simulink model "example1"  (R2024b)
settings: Solver=FixedStepAuto  StartTime=0.0  StopTime=20  FixedStep=0.001  RelTol=1e-3
(part 1 of 3)
settings Model: Creator=aqx  LastModifiedBy=aqx
settings ModelReferenceCC: EnableRefExpFcnMdlSchedulingChecks=on
settings RTWCC: GPUComputeCapability=3.5

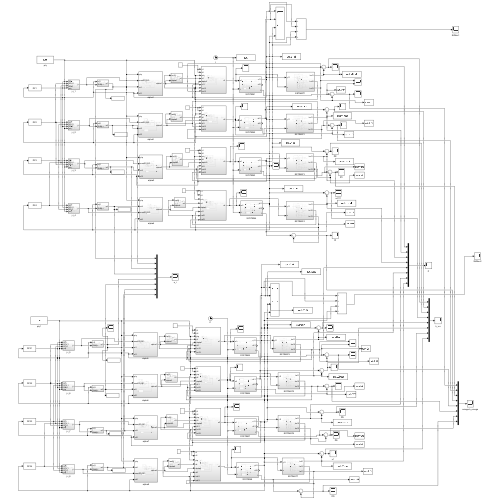
[thumbnail: Simulink's stored preview of the top-level diagram]
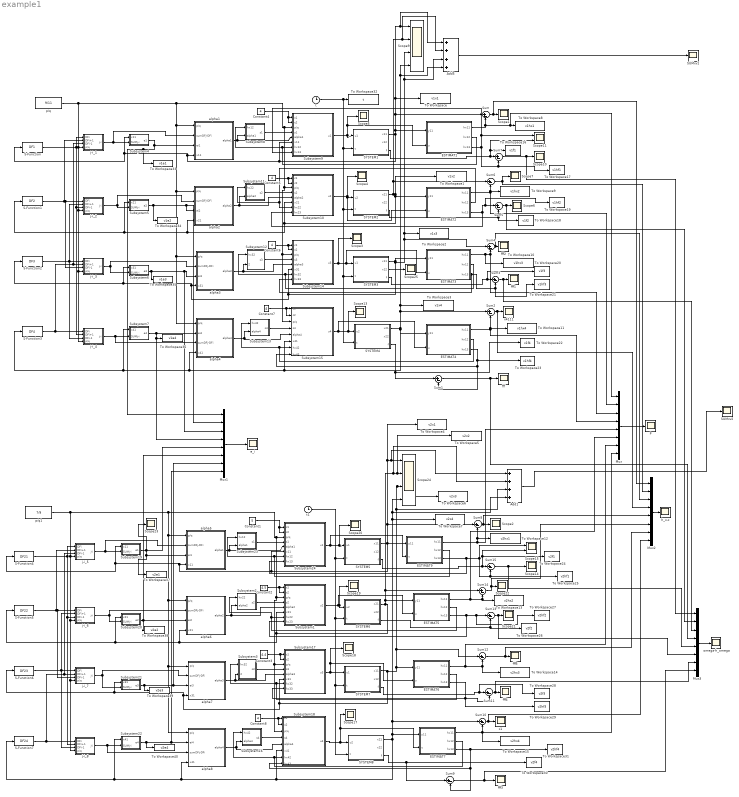
== system example1 ==
  Add1 : Sum  Inputs=4
  Add5 : Sum  Inputs=4
  Constant1 : Constant  Value=5
  Constant2 : Constant  Value=4.5
  Constant3 : Constant  Value=4.4
  Constant{4..8} (5 alike) : Constant  Value=4
  ESTIMAT1 : Subsystem
  ESTIMAT2 : Subsystem
  ESTIMAT3 : Subsystem
  ESTIMAT4 : Subsystem
  ESTIMAT5 : Subsystem
  ESTIMAT6 : Subsystem
  ESTIMAT7 : Subsystem
  ESTIMAT9 : Subsystem
  Mux{,1..3} (4 alike) : Mux  Inputs=8
  P : Scope
  S-Function : S-Function  FunctionName=DF1  SFunctionDeploymentMode=off  EnableBusSupport=off
  S-Function1 : S-Function  FunctionName=DF2  SFunctionDeploymentMode=off  EnableBusSupport=off
  S-Function2 : S-Function  FunctionName=DF3  SFunctionDeploymentMode=off  EnableBusSupport=off
  S-Function3 : S-Function  FunctionName=DF4  SFunctionDeploymentMode=off  EnableBusSupport=off
  S-Function4 : S-Function  FunctionName=DF21  SFunctionDeploymentMode=off  EnableBusSupport=off
  S-Function5 : S-Function  FunctionName=DF22  SFunctionDeploymentMode=off  EnableBusSupport=off
  S-Function6 : S-Function  FunctionName=DF23  SFunctionDeploymentMode=off  EnableBusSupport=off
  S-Function7 : S-Function  FunctionName=DF24  SFunctionDeploymentMode=off  EnableBusSupport=off
  SUMxv1 : Scope
  SUMxv2 : Scope
  SYSTEM1 : Subsystem
  SYSTEM2 : Subsystem
  SYSTEM3 : Subsystem
  SYSTEM4 : Subsystem
  SYSTEM5 : Subsystem
  SYSTEM6 : Subsystem
  SYSTEM7 : Subsystem
  SYSTEM8 : Subsystem
  Scope{1..7,10,13..14,17..23,25} (18 alike) : Scope
  Scope11 : Scope  NumInputPorts=2
  Scope15 : Scope  NumInputPorts=2
  Scope24 : Scope  NumInputPorts=4
  Scope9 : Scope  NumInputPorts=4
  Subsystem1 : Subsystem
  Subsystem10 : Subsystem
  Subsystem11 : Subsystem
  Subsystem12 : Subsystem
  Subsystem13 : Subsystem
  Subsystem14 : Subsystem
  Subsystem15 : Subsystem
  Subsystem16 : Subsystem
  Subsystem17 : Subsystem
  Subsystem18 : Subsystem
  Subsystem19 : Subsystem
  Subsystem2 : Subsystem
  Subsystem20 : Subsystem
  Subsystem21 : Subsystem
  Subsystem22 : Subsystem
  Subsystem23 : Subsystem
  Subsystem24 : Subsystem
  Subsystem3 : Subsystem
  Subsystem4 : Subsystem
  Subsystem5 : Subsystem
  Subsystem6 : Subsystem
  Subsystem7 : Subsystem
  Subsystem8 : Subsystem
  Subsystem9 : Subsystem
  Sum{,1..15} (16 alike) : Sum  Inputs=|+-
  To Workspace : ToWorkspace  VariableName=v1x1  SampleTime=-1
  To Workspace1 : ToWorkspace  VariableName=v1x2  SampleTime=-1
  To Workspace10 : ToWorkspace  VariableName=v1hx3  SampleTime=-1
  To Workspace11 : ToWorkspace  VariableName=v1hx4  SampleTime=-1
  To Workspace12 : ToWorkspace  VariableName=v2hx1  SampleTime=-1
  To Workspace13 : ToWorkspace  VariableName=v2hx2  SampleTime=-1
  To Workspace14 : ToWorkspace  VariableName=v2hx3  SampleTime=-1
  To Workspace15 : ToWorkspace  VariableName=v2hx4  SampleTime=-1
  To Workspace16 : ToWorkspace  VariableName=v1f1  SampleTime=-1
  To Workspace17 : ToWorkspace  VariableName=v1hf1  SampleTime=-1
  To Workspace18 : ToWorkspace  VariableName=v1f2  SampleTime=-1
  To Workspace19 : ToWorkspace  VariableName=v1hf2  SampleTime=-1
  To Workspace2 : ToWorkspace  VariableName=v1x3  SampleTime=-1
  To Workspace20 : ToWorkspace  VariableName=v1f3  SampleTime=-1
  To Workspace21 : ToWorkspace  VariableName=v1hf3  SampleTime=-1
  To Workspace22 : ToWorkspace  VariableName=v1f4  SampleTime=-1
  To Workspace23 : ToWorkspace  VariableName=v1hf4  SampleTime=-1
  To Workspace24 : ToWorkspace  VariableName=v2f1  SampleTime=-1
  To Workspace25 : ToWorkspace  VariableName=v2hf1  SampleTime=-1
  To Workspace26 : ToWorkspace  VariableName=v2f2  SampleTime=-1
  To Workspace27 : ToWorkspace  VariableName=v2hf2  SampleTime=-1
  To Workspace28 : ToWorkspace  VariableName=v2f3  SampleTime=-1
  To Workspace29 : ToWorkspace  VariableName=v2hf3  SampleTime=-1
  To Workspace3 : ToWorkspace  VariableName=v1x4  SampleTime=-1
  To Workspace30 : ToWorkspace  VariableName=v2f4  SampleTime=-1
  To Workspace31 : ToWorkspace  VariableName=v2hf4  SampleTime=-1
  To Workspace32 : ToWorkspace  VariableName=t  SampleTime=-1
  To Workspace33 : ToWorkspace  VariableName=v1e1  SampleTime=-1
  To Workspace34 : ToWorkspace  VariableName=v1e2  SampleTime=-1
  To Workspace35 : ToWorkspace  VariableName=v1e3  SampleTime=-1
  To Workspace36 : ToWorkspace  VariableName=v1e4  SampleTime=-1
  To Workspace37 : ToWorkspace  VariableName=v2e1  SampleTime=-1
  To Workspace38 : ToWorkspace  VariableName=v2e2  SampleTime=-1
  To Workspace39 : ToWorkspace  VariableName=v2e3  SampleTime=-1
  To Workspace4 : ToWorkspace  VariableName=v2x1  SampleTime=-1
  To Workspace40 : ToWorkspace  VariableName=v2e4  SampleTime=-1
  To Workspace5 : ToWorkspace  VariableName=v2x2  SampleTime=-1
  To Workspace6 : ToWorkspace  VariableName=v2x3  SampleTime=-1
  To Workspace7 : ToWorkspace  VariableName=v2x4  SampleTime=-1
  To Workspace8 : ToWorkspace  VariableName=v1hx1  SampleTime=-1
  To Workspace9 : ToWorkspace  VariableName=v1hx2  SampleTime=-1
  alpha1 : Subsystem
  alpha2 : Subsystem
  alpha3 : Subsystem
  alpha4 : Subsystem
  alpha5 : Subsystem
  alpha6 : Subsystem
  alpha7 : Subsystem
  alpha8 : Subsystem
  e_i : Scope
  fff{,1..5} (6 alike) : Scope
  h_x-x : Scope
  j-i_1 : Subsystem
  j-i_2 : Subsystem
  j-i_3 : Subsystem
  j-i_4 : Subsystem
  j-i_5 : Subsystem
  j-i_6 : Subsystem
  j-i_7 : Subsystem
  j-i_8 : Subsystem
  omega-h_omega : Scope
  p/q : Constant  Value=9/11
  p/q1 : Constant  Value=7/9
  t : Clock
  t1 : Clock
  x1 : Scope
  x4111 : Scope
  wires:
  S-Function/1 -> j-i_4/2(DFi+1), j-i_2/3(DFi-1), j-i_1/1(DFi)
  S-Function1/1 -> j-i_3/3(DFi-1), j-i_2/1(DFi), j-i_1/2(DFi+1)
  S-Function3/1 -> j-i_3/2(DFi+1), j-i_1/3(DFi-1), j-i_4/1(DFi)
  S-Function2/1 -> j-i_2/2(DFi+1), j-i_4/3(DFi-1), j-i_3/1(DFi)
  j-i_1/1(j-i) -> Subsystem4/2(SUMj-i), alpha1/2(sumDFj-DFi)
  j-i_2/1(j-i) -> alpha2/2(sumDFj-DFi), Subsystem5/2(SUMj-i)
  j-i_3/1(j-i) -> Subsystem6/2(SUMj-i), alpha3/2(sumDFj-DFi)
  j-i_4/1(j-i) -> alpha4/3(sumDFj-DFi), Subsystem7/2(SUMj-i)
  Subsystem4/1(e1) -> Mux1/1, To Workspace33/1, alpha1/3(ei1)
  Subsystem5/1(e2) -> To Workspace34/1, Mux1/2, alpha2/3(ei2)
  Subsystem6/1(e3) -> To Workspace35/1, Mux1/3, alpha3/3(ei3)
  Subsystem7/1(e4) -> Mux1/4, To Workspace36/1, alpha4/2(ei4)
  p/q/1 -> j-i_4/4(p/q), j-i_3/4(p/q), j-i_2/4(p/q), j-i_1/4(p/q), alpha4/1(p/q), alpha3/1(p/q), alpha2/1(p/q), alpha1/1(p/q), Subsystem15/3(p/q), Subsystem14/3(p/q), Subsystem10/3(p/q), Subsystem9/3(p/q)
  alpha1/1(alpha1) -> Subsystem8/2(alpha1), Subsystem9/5(alpha1)
  Subsystem8/1(s1) -> Subsystem9/4(s1)
  alpha2/1(alpha2) -> Subsystem10/5(alpha2), Subsystem11/2(alpha2)
  Subsystem11/1(s2) -> Subsystem10/4(s2)
  alpha3/1(alpha3) -> Subsystem12/2(alpha3), Subsystem14/5(alpha3)
  alpha4/1(alpha4) -> Subsystem15/5(alpha4), Subsystem13/2(alpha4)
  Subsystem12/1(s3) -> Subsystem14/4(s3)
  Subsystem13/1(s4) -> Subsystem15/4(s4)
  Subsystem14/1(u3) -> ESTIMAT3/2(u), SYSTEM3/1(u1), Scope3/1
  Subsystem15/1(u4) -> ESTIMAT4/2(u), Scope13/1, SYSTEM4/1(u2)
  Constant4/1 -> Subsystem9/2(c2), Subsystem9/1(c1)
  Subsystem9/1(u1) -> ESTIMAT1/2(u), Scope5/1, SYSTEM1/1(u1)
  Subsystem10/1(u2) -> ESTIMAT2/2(u), SYSTEM2/1(u2), Scope4/1
  Constant5/1 -> Subsystem10/2(c2), Subsystem10/1(c1)
  Constant6/1 -> Subsystem14/2(c2), Subsystem14/1(c1)
  Constant7/1 -> Subsystem15/2(c2), Subsystem15/1(c1)
  SYSTEM1/1(x11) -> To Workspace/1, Add5/1, Scope9/1, Sum/1, ESTIMAT1/1(y11), S-Function/1, Subsystem4/1(x11), alpha1/4(x11), Subsystem9/6(x11)
  SYSTEM2/1(x21) -> Add5/2, Scope9/2, Sum6/1, ESTIMAT2/1(y11), S-Function1/1, Subsystem5/1(x21), alpha2/4(x21), Subsystem10/6(x21), To Workspace1/1
  SYSTEM3/1(x11) -> Subsystem14/6(x31), S-Function2/1, Subsystem6/1(x31), alpha3/4(x31), To Workspace2/1, Scope9/3, Add5/3, Sum4/1, ESTIMAT3/1(y11)
  SYSTEM4/1(x21) -> ESTIMAT4/1(y11), Subsystem15/6(x41), S-Function3/1, Subsystem7/1(x41), alpha4/4(x41), Scope9/4, Add5/4, To Workspace3/1, Sum2/1
  Sum/1 -> Mux2/1, Scope1/1
  SYSTEM4/3(f) -> Sum1/1, To Workspace22/1
  Sum1/1 -> Mux3/4, fff/1
  Sum2/1 -> Mux2/4, x4111/1
  SYSTEM3/3(f) -> To Workspace20/1, Sum3/1
  Sum3/1 -> Mux3/3, fff1/1
  Sum4/1 -> Mux2/3, fff2/1
  SYSTEM2/3(f) -> To Workspace18/1, Sum5/2
  Sum5/1 -> Mux3/2, Scope6/1
  Sum6/1 -> Mux2/2, Scope7/1
  SYSTEM1/3(f) -> Scope11/2, To Workspace16/1, Sum7/1
  Sum7/1 -> Mux3/1, Scope10/1
  Add5/1 -> SUMxv1/1
  Subsystem20/1(e2) -> To Workspace38/1, Mux1/6, alpha6/3(ei2)
  Subsystem19/1(e1) -> Mux1/5, To Workspace37/1, alpha5/3(ei1), Scope23/1
  Subsystem22/1(e4) -> Mux1/8, alpha8/2(ei4), To Workspace40/1
  S-Function4/1 -> j-i_8/2(DFi+1), j-i_6/3(DFi-1), j-i_5/1(DFi)
  S-Function5/1 -> j-i_7/3(DFi-1), j-i_6/1(DFi), j-i_5/2(DFi+1)
  Sum11/1 -> Mux3/7, fff4/1
  SYSTEM7/3(f) -> To Workspace28/1, Sum11/1
  Subsystem16/1(s4) -> Subsystem18/4(s4)
  ESTIMAT7/2(hx12) -> Subsystem16/1(hx42), Subsystem18/7(hx42)
  ESTIMAT7/1(hx11) -> Mux/8, To Workspace15/1, Sum10/2
  S-Function7/1 -> j-i_7/2(DFi+1), j-i_5/3(DFi-1), j-i_8/1(DFi)
  SYSTEM8/3(f) -> To Workspace30/1, Sum9/1
  j-i_6/1(j-i) -> alpha6/2(sumDFj-DFi), Subsystem20/2(SUMj-i)
  ESTIMAT9/1(hx11) -> Mux/5, Sum8/2, To Workspace12/1
  alpha5/1(alpha1) -> Subsystem23/2(alpha1), Subsystem24/5(alpha1)
  Sum8/1 -> Mux2/5, Scope2/1
  ESTIMAT7/3(hx13) -> Sum9/2, Subsystem18/8(hx43), To Workspace31/1
  Constant1/1 -> Subsystem24/2(c2), Subsystem24/1(c1)
  ESTIMAT6/3(hx13) -> Sum11/2, Subsystem17/8(hx33), To Workspace29/1
  SYSTEM7/1(x11) -> ESTIMAT6/1(y11), To Workspace6/1, Scope24/3, Add1/3, Sum12/1, Subsystem17/6(x31), S-Function6/1, Subsystem21/1(x31), alpha7/4(x31)
  ESTIMAT6/2(hx12) -> Subsystem3/1(hx32), Subsystem17/7(hx32)
  ESTIMAT5/2(hx12) -> Subsystem2/1(hx22), Subsystem1/7(hx22)
  Subsystem21/1(e3) -> Mux1/7, alpha7/3(ei3), To Workspace39/1
  Constant3/1 -> Subsystem17/2(c2), Subsystem17/1(c1)
  SYSTEM5/1(x11) -> ESTIMAT9/1(y11), To Workspace4/1, Add1/1, Scope24/1, Sum8/1, S-Function4/1, Subsystem19/1(x11), alpha5/4(x11), Subsystem24/6(x11)
  t1/1 -> SYSTEM8/2(t), SYSTEM7/2(t), SYSTEM6/2(t), SYSTEM5/2(t)
  SYSTEM6/1(x21) -> ESTIMAT5/1(y11), Add1/2, To Workspace5/1, Scope24/2, Sum14/1, S-Function5/1, Subsystem20/1(x21), alpha6/4(x21), Subsystem1/6(x21)
  Constant8/1 -> Subsystem18/2(c2), Subsystem18/1(c1)
  Constant2/1 -> Subsystem1/2(c2), Subsystem1/1(c1)
  Subsystem18/1(u4) -> ESTIMAT7/2(u), Scope17/1, SYSTEM8/1(u2)
  j-i_8/1(j-i) -> alpha8/3(sumDFj-DFi), Subsystem22/2(SUMj-i)
  j-i_5/1(j-i) -> Subsystem19/2(SUMj-i), alpha5/2(sumDFj-DFi)
  Subsystem17/1(u3) -> SYSTEM7/1(u1), ESTIMAT6/2(u), Scope18/1
  Subsystem3/1(s3) -> Subsystem17/4(s3)
  alpha8/1(alpha4) -> Subsystem18/5(alpha4), Subsystem16/2(alpha4)
  alpha7/1(alpha3) -> Subsystem3/2(alpha3), Subsystem17/5(alpha3)
  alpha6/1(alpha2) -> Subsystem1/5(alpha2), Subsystem2/2(alpha2)
  p/q1/1 -> j-i_8/4(p/q), j-i_7/4(p/q), j-i_6/4(p/q), j-i_5/4(p/q), alpha8/1(p/q), alpha7/1(p/q), alpha6/1(p/q), alpha5/1(p/q), Subsystem18/3(p/q), Subsystem17/3(p/q), Subsystem1/3(p/q), Subsystem24/3(p/q)
  ESTIMAT6/1(hx11) -> Mux/7, To Workspace14/1, Sum12/2
  Subsystem2/1(s2) -> Subsystem1/4(s2)
  Sum9/1 -> Mux3/8, fff3/1
  SYSTEM5/3(f) -> Scope15/2, To Workspace24/1, Sum15/1
  j-i_7/1(j-i) -> Subsystem21/2(SUMj-i), alpha7/2(sumDFj-DFi)
  Sum10/1 -> Mux2/8, x1/1
  Sum15/1 -> Mux3/5, Scope14/1
  SYSTEM8/1(x21) -> ESTIMAT7/1(y11), Scope24/4, Add1/4, To Workspace7/1, Sum10/1, Subsystem18/6(x41), S-Function7/1, Subsystem22/1(x41), alpha8/4(x41)
  Add1/1 -> SUMxv2/1
  Sum12/1 -> Mux2/7, fff5/1
  ESTIMAT9/3(hx13) -> Subsystem24/8(hx13), To Workspace25/1, Sum15/2, Scope15/1
  S-Function6/1 -> j-i_6/2(DFi+1), j-i_8/3(DFi-1), j-i_7/1(DFi)
  Sum13/1 -> Mux3/6, Scope21/1
  Subsystem1/1(u2) -> ESTIMAT5/2(u), Scope19/1, SYSTEM6/1(u2)
  Subsystem24/1(u1) -> ESTIMAT9/2(u), SYSTEM5/1(u1), Scope20/1
  Sum14/1 -> Mux2/6, Scope22/1
  Subsystem23/1(s1) -> Subsystem24/4(s1)
  ESTIMAT5/1(hx11) -> Mux/6, To Workspace13/1, Sum14/2
  ESTIMAT5/3(hx13) -> To Workspace27/1, Sum13/1, Subsystem1/8(hx23)
  SYSTEM6/3(f) -> Sum13/2, To Workspace26/1
  ESTIMAT9/2(hx12) -> Subsystem23/1(hx12), Subsystem24/7(hx12)
  t/1 -> To Workspace32/1, SYSTEM4/2(t), SYSTEM3/2(t), SYSTEM2/2(t), SYSTEM1/2(t)
  ESTIMAT1/1(hx11) -> Sum/2, Mux/1, To Workspace8/1
  ESTIMAT1/3(hx13) -> Subsystem9/8(hx13), Scope11/1, To Workspace17/1, Sum7/2
  ESTIMAT1/2(hx12) -> Subsystem8/1(hx12), Subsystem9/7(hx12)
  ESTIMAT2/1(hx11) -> Mux/2, To Workspace9/1, Sum6/2
  ESTIMAT2/3(hx13) -> Subsystem10/8(hx23), To Workspace19/1, Sum5/1
  ESTIMAT2/2(hx12) -> Subsystem10/7(hx22), Subsystem11/1(hx22)
  ESTIMAT3/1(hx11) -> To Workspace10/1, Mux/3, Sum4/2
  ESTIMAT3/3(hx13) -> Subsystem14/8(hx33), To Workspace21/1, Sum3/2
  ESTIMAT3/2(hx12) -> Subsystem12/1(hx32), Subsystem14/7(hx32)
  ESTIMAT4/1(hx11) -> Sum2/2, To Workspace11/1, Mux/4
  ESTIMAT4/3(hx13) -> To Workspace23/1, Subsystem15/8(hx43), Sum1/2
  ESTIMAT4/2(hx12) -> Subsystem13/1(hx42), Subsystem15/7(hx42)
  SYSTEM3/2(x12) -> Scope25/1
  Mux/1 -> P/1
  Mux1/1 -> e_i/1
  Mux2/1 -> h_x-x/1
  Mux3/1 -> omega-h_omega/1

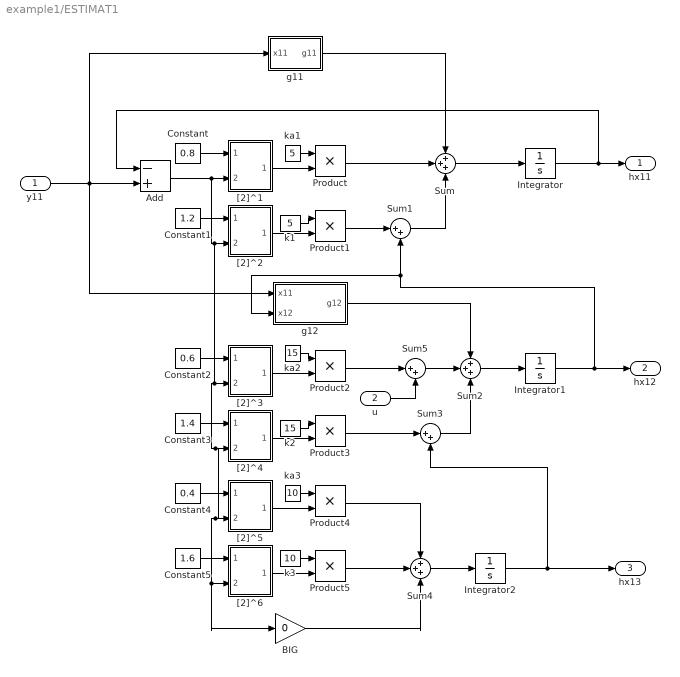
== system example1/ESTIMAT1 ==
  y11 : Inport
  u : Inport  Port=2
  Add : Sum  Inputs=-+
  BIG : Gain  Gain=0
  Constant : Constant  Value=0.8
  Constant1 : Constant  Value=1.2
  Constant2 : Constant  Value=0.6
  Constant3 : Constant  Value=1.4
  Constant4 : Constant  Value=0.4
  Constant5 : Constant  Value=1.6
  Integrator : Integrator  InitialCondition=1
  Integrator1 : Integrator  InitialCondition=1
  Integrator2 : Integrator  InitialCondition=1
  Product{,1..5} (6 alike) : Product
  Sum : Sum  Inputs=3
  Sum1 : Sum  Inputs=|++
  Sum2 : Sum  Inputs=3
  Sum3 : Sum  Inputs=|++
  Sum4 : Sum  Inputs=3
  Sum5 : Sum  Inputs=|++
  "[2]^1" : Subsystem
  "[2]^2" : Subsystem
  "[2]^3" : Subsystem
  "[2]^4" : Subsystem
  "[2]^5" : Subsystem
  "[2]^6" : Subsystem
  g11 : Subsystem
  g12 : Subsystem
  k1 : Constant  Value=5
  k2 : Constant  Value=15
  k3 : Constant  Value=10
  ka1 : Constant  Value=5
  ka2 : Constant  Value=15
  ka3 : Constant  Value=10
  hx11 : Outport
  hx12 : Outport  Port=2
  hx13 : Outport  Port=3
  wires:
  Integrator/1 -> Add/1, hx11/1
  Sum1/1 -> Sum/3
  Sum/1 -> Integrator/1
  Integrator1/1 -> g12/2(x12), Sum1/2, hx12/1
  y11/1 -> g12/1(x11), g11/1(x11), Add/2
  "[2]^1"/1(Out1) -> Product/2
  "[2]^2"/1(Out1) -> Product1/2
  ka1/1 -> Product/1
  k1/1 -> Product1/1
  g11/1(g11) -> Sum/1
  Product/1 -> Sum/2
  Product1/1 -> Sum1/1
  Sum2/1 -> Integrator1/1
  Sum3/1 -> Sum2/3
  Integrator2/1 -> hx13/1, Sum3/2
  g12/1(g12) -> Sum2/1
  ka2/1 -> Product2/1
  k2/1 -> Product3/1
  "[2]^4"/1(Out1) -> Product3/2
  "[2]^3"/1(Out1) -> Product2/2
  Product3/1 -> Sum3/1
  Sum4/1 -> Integrator2/1
  k3/1 -> Product5/1
  "[2]^6"/1(Out1) -> Product5/2
  ka3/1 -> Product4/1
  Add/1 -> BIG/1, "[2]^6"/2(In2), "[2]^5"/2(In2), "[2]^4"/2(In2), "[2]^3"/2(In2), "[2]^2"/2(In2), "[2]^1"/2(In2)
  "[2]^5"/1(Out1) -> Product4/2
  Product5/1 -> Sum4/2
  Product4/1 -> Sum4/1
  BIG/1 -> Sum4/3
  Product2/1 -> Sum5/1
  Sum5/1 -> Sum2/2
  u/1 -> Sum5/2
  Constant/1 -> "[2]^1"/1(In1)
  Constant1/1 -> "[2]^2"/1(beta1)
  Constant2/1 -> "[2]^3"/1(In1)
  Constant3/1 -> "[2]^4"/1(beta1)
  Constant4/1 -> "[2]^5"/1(In1)
  Constant5/1 -> "[2]^6"/1(beta1)

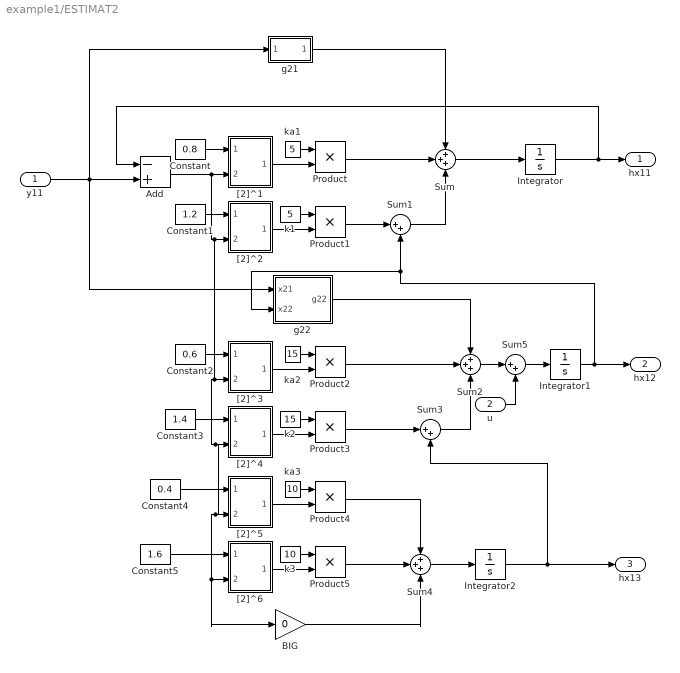
== system example1/ESTIMAT2 ==
  y11 : Inport
  u : Inport  Port=2
  Add : Sum  Inputs=-+
  BIG : Gain  Gain=0
  Constant : Constant  Value=0.8
  Constant1 : Constant  Value=1.2
  Constant2 : Constant  Value=0.6
  Constant3 : Constant  Value=1.4
  Constant4 : Constant  Value=0.4
  Constant5 : Constant  Value=1.6
  Integrator : Integrator  InitialCondition=3
  Integrator1 : Integrator  InitialCondition=1
  Integrator2 : Integrator  InitialCondition=1
  Product{,1..5} (6 alike) : Product
  Sum : Sum  Inputs=3
  Sum1 : Sum  Inputs=|++
  Sum2 : Sum  Inputs=3
  Sum3 : Sum  Inputs=|++
  Sum4 : Sum  Inputs=3
  Sum5 : Sum  Inputs=|++
  "[2]^1" : Subsystem
  "[2]^2" : Subsystem
  "[2]^3" : Subsystem
  "[2]^4" : Subsystem
  "[2]^5" : Subsystem
  "[2]^6" : Subsystem
  g21 : Subsystem
  g22 : Subsystem
  k1 : Constant  Value=5
  k2 : Constant  Value=15
  k3 : Constant  Value=10
  ka1 : Constant  Value=5
  ka2 : Constant  Value=15
  ka3 : Constant  Value=10
  hx11 : Outport
  hx12 : Outport  Port=2
  hx13 : Outport  Port=3
  wires:
  Integrator/1 -> Add/1, hx11/1
  Sum1/1 -> Sum/3
  Sum/1 -> Integrator/1
  Integrator1/1 -> g22/2(x22), Sum1/2, hx12/1
  y11/1 -> g22/1(x21), g21/1(x21), Add/2
  "[2]^1"/1(Out1) -> Product/2
  "[2]^2"/1(Out1) -> Product1/2
  ka1/1 -> Product/1
  k1/1 -> Product1/1
  g21/1(g21) -> Sum/1
  Product/1 -> Sum/2
  Product1/1 -> Sum1/1
  Sum3/1 -> Sum2/3
  Integrator2/1 -> hx13/1, Sum3/2
  g22/1(g22) -> Sum2/1
  ka2/1 -> Product2/1
  k2/1 -> Product3/1
  "[2]^4"/1(Out1) -> Product3/2
  "[2]^3"/1(Out1) -> Product2/2
  Product2/1 -> Sum2/2
  Product3/1 -> Sum3/1
  Sum4/1 -> Integrator2/1
  k3/1 -> Product5/1
  "[2]^6"/1(Out1) -> Product5/2
  ka3/1 -> Product4/1
  Add/1 -> BIG/1, "[2]^6"/2(In2), "[2]^5"/2(In2), "[2]^4"/2(In2), "[2]^3"/2(In2), "[2]^2"/2(In2), "[2]^1"/2(In2)
  "[2]^5"/1(Out1) -> Product4/2
  Product5/1 -> Sum4/2
  Product4/1 -> Sum4/1
  BIG/1 -> Sum4/3
  Sum2/1 -> Sum5/1
  Sum5/1 -> Integrator1/1
  u/1 -> Sum5/2
  Constant/1 -> "[2]^1"/1(In1)
  Constant1/1 -> "[2]^2"/1(beta1)
  Constant2/1 -> "[2]^3"/1(In1)
  Constant3/1 -> "[2]^4"/1(beta1)
  Constant4/1 -> "[2]^5"/1(In1)
  Constant5/1 -> "[2]^6"/1(beta1)

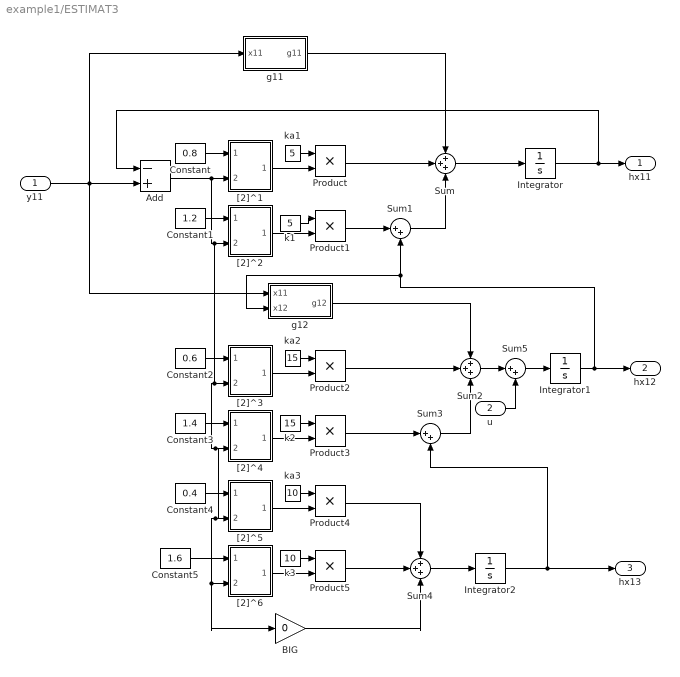
== system example1/ESTIMAT3 ==
  y11 : Inport
  u : Inport  Port=2
  Add : Sum  Inputs=-+
  BIG : Gain  Gain=0
  Constant : Constant  Value=0.8
  Constant1 : Constant  Value=1.2
  Constant2 : Constant  Value=0.6
  Constant3 : Constant  Value=1.4
  Constant4 : Constant  Value=0.4
  Constant5 : Constant  Value=1.6
  Integrator : Integrator  InitialCondition=1
  Integrator1 : Integrator  InitialCondition=1
  Integrator2 : Integrator  InitialCondition=1
  Product{,1..5} (6 alike) : Product
  Sum : Sum  Inputs=3
  Sum1 : Sum  Inputs=|++
  Sum2 : Sum  Inputs=3
  Sum3 : Sum  Inputs=|++
  Sum4 : Sum  Inputs=3
  Sum5 : Sum  Inputs=|++
  "[2]^1" : Subsystem
  "[2]^2" : Subsystem
  "[2]^3" : Subsystem
  "[2]^4" : Subsystem
  "[2]^5" : Subsystem
  "[2]^6" : Subsystem
  g11 : Subsystem
  g12 : Subsystem
  k1 : Constant  Value=5
  k2 : Constant  Value=15
  k3 : Constant  Value=10
  ka1 : Constant  Value=5
  ka2 : Constant  Value=15
  ka3 : Constant  Value=10
  hx11 : Outport
  hx12 : Outport  Port=2
  hx13 : Outport  Port=3
  wires:
  Integrator/1 -> Add/1, hx11/1
  Sum1/1 -> Sum/3
  Sum/1 -> Integrator/1
  Integrator1/1 -> g12/2(x12), Sum1/2, hx12/1
  y11/1 -> g12/1(x11), g11/1(x11), Add/2
  "[2]^1"/1(Out1) -> Product/2
  "[2]^2"/1(Out1) -> Product1/2
  ka1/1 -> Product/1
  k1/1 -> Product1/1
  g11/1(g11) -> Sum/1
  Product/1 -> Sum/2
  Product1/1 -> Sum1/1
  Sum3/1 -> Sum2/3
  Integrator2/1 -> hx13/1, Sum3/2
  g12/1(g12) -> Sum2/1
  ka2/1 -> Product2/1
  k2/1 -> Product3/1
  "[2]^4"/1(Out1) -> Product3/2
  "[2]^3"/1(Out1) -> Product2/2
  Product2/1 -> Sum2/2
  Product3/1 -> Sum3/1
  Sum4/1 -> Integrator2/1
  k3/1 -> Product5/1
  "[2]^6"/1(Out1) -> Product5/2
  ka3/1 -> Product4/1
  Add/1 -> BIG/1, "[2]^6"/2(In2), "[2]^5"/2(In2), "[2]^4"/2(In2), "[2]^3"/2(In2), "[2]^2"/2(In2), "[2]^1"/2(In2)
  "[2]^5"/1(Out1) -> Product4/2
  Product5/1 -> Sum4/2
  Product4/1 -> Sum4/1
  BIG/1 -> Sum4/3
  Sum2/1 -> Sum5/1
  Sum5/1 -> Integrator1/1
  u/1 -> Sum5/2
  Constant/1 -> "[2]^1"/1(In1)
  Constant1/1 -> "[2]^2"/1(beta1)
  Constant2/1 -> "[2]^3"/1(In1)
  Constant3/1 -> "[2]^4"/1(beta1)
  Constant4/1 -> "[2]^5"/1(In1)
  Constant5/1 -> "[2]^6"/1(beta1)

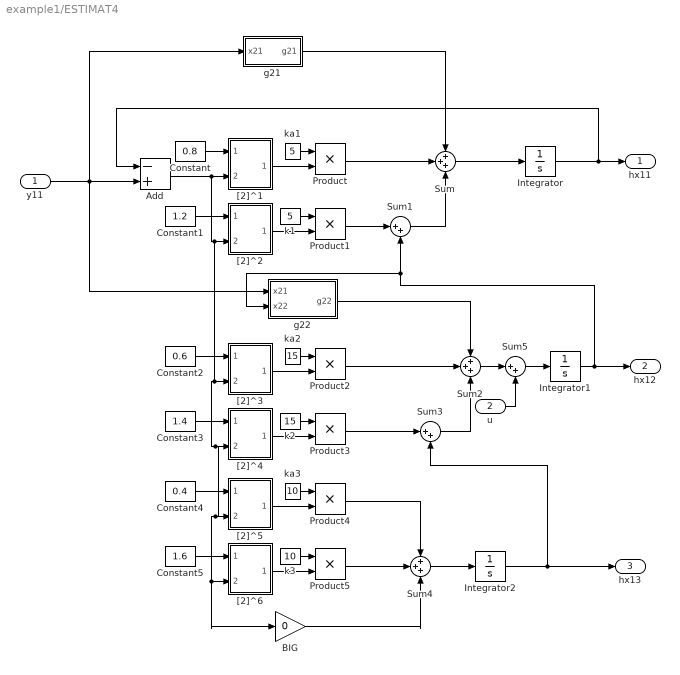
== system example1/ESTIMAT4 ==
  y11 : Inport
  u : Inport  Port=2
  Add : Sum  Inputs=-+
  BIG : Gain  Gain=0
  Constant : Constant  Value=0.8
  Constant1 : Constant  Value=1.2
  Constant2 : Constant  Value=0.6
  Constant3 : Constant  Value=1.4
  Constant4 : Constant  Value=0.4
  Constant5 : Constant  Value=1.6
  Integrator : Integrator  InitialCondition=5
  Integrator1 : Integrator  InitialCondition=1
  Integrator2 : Integrator  InitialCondition=1
  Product{,1..5} (6 alike) : Product
  Sum : Sum  Inputs=3
  Sum1 : Sum  Inputs=|++
  Sum2 : Sum  Inputs=3
  Sum3 : Sum  Inputs=|++
  Sum4 : Sum  Inputs=3
  Sum5 : Sum  Inputs=|++
  "[2]^1" : Subsystem
  "[2]^2" : Subsystem
  "[2]^3" : Subsystem
  "[2]^4" : Subsystem
  "[2]^5" : Subsystem
  "[2]^6" : Subsystem
  g21 : Subsystem
  g22 : Subsystem
  k1 : Constant  Value=5
  k2 : Constant  Value=15
  k3 : Constant  Value=10
  ka1 : Constant  Value=5
  ka2 : Constant  Value=15
  ka3 : Constant  Value=10
  hx11 : Outport
  hx12 : Outport  Port=2
  hx13 : Outport  Port=3
  wires:
  Integrator/1 -> Add/1, hx11/1
  Sum1/1 -> Sum/3
  Sum/1 -> Integrator/1
  Integrator1/1 -> g22/2(x22), Sum1/2, hx12/1
  y11/1 -> g22/1(x21), g21/1(x21), Add/2
  "[2]^1"/1(Out1) -> Product/2
  "[2]^2"/1(Out1) -> Product1/2
  ka1/1 -> Product/1
  k1/1 -> Product1/1
  g21/1(g21) -> Sum/1
  Product/1 -> Sum/2
  Product1/1 -> Sum1/1
  Sum3/1 -> Sum2/3
  Integrator2/1 -> hx13/1, Sum3/2
  g22/1(g22) -> Sum2/1
  ka2/1 -> Product2/1
  k2/1 -> Product3/1
  "[2]^4"/1(Out1) -> Product3/2
  "[2]^3"/1(Out1) -> Product2/2
  Product2/1 -> Sum2/2
  Product3/1 -> Sum3/1
  Sum4/1 -> Integrator2/1
  k3/1 -> Product5/1
  "[2]^6"/1(Out1) -> Product5/2
  ka3/1 -> Product4/1
  Add/1 -> BIG/1, "[2]^6"/2(In2), "[2]^5"/2(In2), "[2]^4"/2(In2), "[2]^3"/2(In2), "[2]^2"/2(In2), "[2]^1"/2(In2)
  "[2]^5"/1(Out1) -> Product4/2
  Product5/1 -> Sum4/2
  Product4/1 -> Sum4/1
  BIG/1 -> Sum4/3
  Sum2/1 -> Sum5/1
  Sum5/1 -> Integrator1/1
  u/1 -> Sum5/2
  Constant/1 -> "[2]^1"/1(In1)
  Constant1/1 -> "[2]^2"/1(beta1)
  Constant2/1 -> "[2]^3"/1(In1)
  Constant3/1 -> "[2]^4"/1(beta1)
  Constant4/1 -> "[2]^5"/1(In1)
  Constant5/1 -> "[2]^6"/1(beta1)

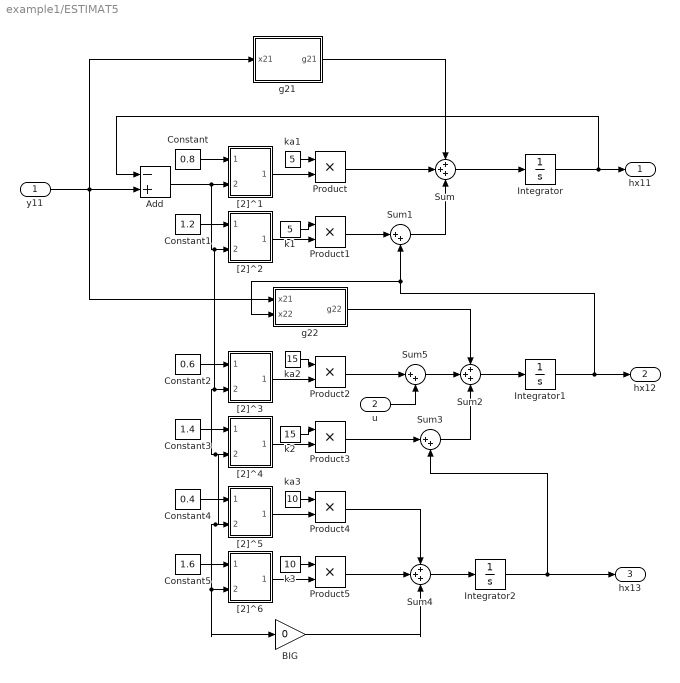
== system example1/ESTIMAT5 ==
  y11 : Inport
  u : Inport  Port=2
  Add : Sum  Inputs=-+
  BIG : Gain  Gain=0
  Constant : Constant  Value=0.8
  Constant1 : Constant  Value=1.2
  Constant2 : Constant  Value=0.6
  Constant3 : Constant  Value=1.4
  Constant4 : Constant  Value=0.4
  Constant5 : Constant  Value=1.6
  Integrator : Integrator  InitialCondition=1
  Integrator1 : Integrator  InitialCondition=1
  Integrator2 : Integrator  InitialCondition=1
  Product{,1..5} (6 alike) : Product
  Sum : Sum  Inputs=3
  Sum1 : Sum  Inputs=|++
  Sum2 : Sum  Inputs=3
  Sum3 : Sum  Inputs=|++
  Sum4 : Sum  Inputs=3
  Sum5 : Sum  Inputs=|++
  "[2]^1" : Subsystem
  "[2]^2" : Subsystem
  "[2]^3" : Subsystem
  "[2]^4" : Subsystem
  "[2]^5" : Subsystem
  "[2]^6" : Subsystem
  g21 : Subsystem
  g22 : Subsystem
  k1 : Constant  Value=5
  k2 : Constant  Value=15
  k3 : Constant  Value=10
  ka1 : Constant  Value=5
  ka2 : Constant  Value=15
  ka3 : Constant  Value=10
  hx11 : Outport
  hx12 : Outport  Port=2
  hx13 : Outport  Port=3
  wires:
  Integrator/1 -> Add/1, hx11/1
  Sum1/1 -> Sum/3
  Sum/1 -> Integrator/1
  Integrator1/1 -> g22/2(x22), Sum1/2, hx12/1
  y11/1 -> g22/1(x21), g21/1(x21), Add/2
  "[2]^1"/1(Out1) -> Product/2
  "[2]^2"/1(Out1) -> Product1/2
  ka1/1 -> Product/1
  k1/1 -> Product1/1
  g21/1(g21) -> Sum/1
  Product/1 -> Sum/2
  Product1/1 -> Sum1/1
  Sum2/1 -> Integrator1/1
  Sum3/1 -> Sum2/3
  Integrator2/1 -> hx13/1, Sum3/2
  g22/1(g22) -> Sum2/1
  ka2/1 -> Product2/1
  k2/1 -> Product3/1
  "[2]^4"/1(Out1) -> Product3/2
  "[2]^3"/1(Out1) -> Product2/2
  Product3/1 -> Sum3/1
  Sum4/1 -> Integrator2/1
  k3/1 -> Product5/1
  "[2]^6"/1(Out1) -> Product5/2
  ka3/1 -> Product4/1
  Add/1 -> BIG/1, "[2]^6"/2(In2), "[2]^5"/2(In2), "[2]^4"/2(In2), "[2]^3"/2(In2), "[2]^2"/2(In2), "[2]^1"/2(In2)
  "[2]^5"/1(Out1) -> Product4/2
  Product5/1 -> Sum4/2
  Product4/1 -> Sum4/1
  BIG/1 -> Sum4/3
  Product2/1 -> Sum5/1
  Sum5/1 -> Sum2/2
  u/1 -> Sum5/2
  Constant/1 -> "[2]^1"/1(In1)
  Constant1/1 -> "[2]^2"/1(beta1)
  Constant2/1 -> "[2]^3"/1(In1)
  Constant3/1 -> "[2]^4"/1(beta1)
  Constant4/1 -> "[2]^5"/1(In1)
  Constant5/1 -> "[2]^6"/1(beta1)

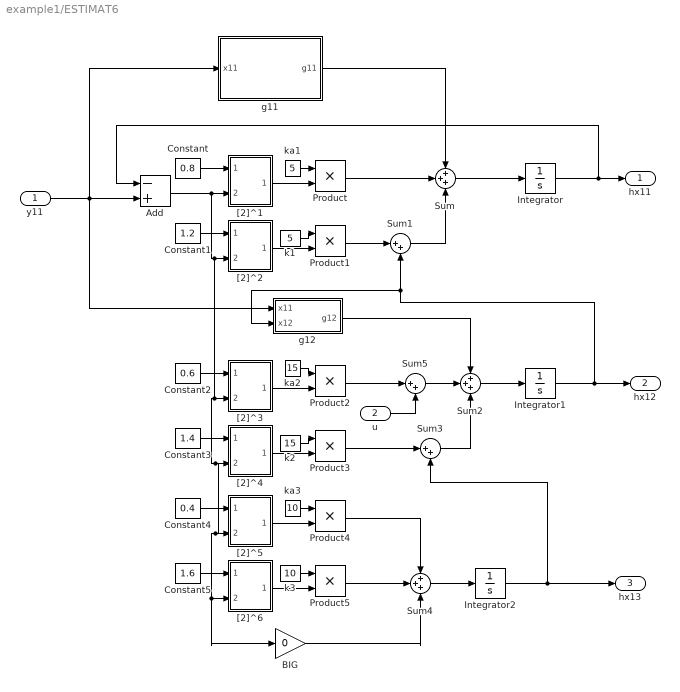
== system example1/ESTIMAT6 ==
  y11 : Inport
  u : Inport  Port=2
  Add : Sum  Inputs=-+
  BIG : Gain  Gain=0
  Constant : Constant  Value=0.8
  Constant1 : Constant  Value=1.2
  Constant2 : Constant  Value=0.6
  Constant3 : Constant  Value=1.4
  Constant4 : Constant  Value=0.4
  Constant5 : Constant  Value=1.6
  Integrator : Integrator  InitialCondition=1
  Integrator1 : Integrator  InitialCondition=1
  Integrator2 : Integrator  InitialCondition=1
  Product{,1..5} (6 alike) : Product
  Sum : Sum  Inputs=3
  Sum1 : Sum  Inputs=|++
  Sum2 : Sum  Inputs=3
  Sum3 : Sum  Inputs=|++
  Sum4 : Sum  Inputs=3
  Sum5 : Sum  Inputs=|++
  "[2]^1" : Subsystem
  "[2]^2" : Subsystem
  "[2]^3" : Subsystem
  "[2]^4" : Subsystem
  "[2]^5" : Subsystem
  "[2]^6" : Subsystem
  g11 : Subsystem
  g12 : Subsystem
  k1 : Constant  Value=5
  k2 : Constant  Value=15
  k3 : Constant  Value=10
  ka1 : Constant  Value=5
  ka2 : Constant  Value=15
  ka3 : Constant  Value=10
  hx11 : Outport
  hx12 : Outport  Port=2
  hx13 : Outport  Port=3
  wires:
  Integrator/1 -> Add/1, hx11/1
  Sum1/1 -> Sum/3
  Sum/1 -> Integrator/1
  Integrator1/1 -> g12/2(x12), Sum1/2, hx12/1
  y11/1 -> g12/1(x11), g11/1(x11), Add/2
  "[2]^1"/1(Out1) -> Product/2
  "[2]^2"/1(Out1) -> Product1/2
  ka1/1 -> Product/1
  k1/1 -> Product1/1
  g11/1(g11) -> Sum/1
  Product/1 -> Sum/2
  Product1/1 -> Sum1/1
  Sum2/1 -> Integrator1/1
  Sum3/1 -> Sum2/3
  Integrator2/1 -> hx13/1, Sum3/2
  g12/1(g12) -> Sum2/1
  ka2/1 -> Product2/1
  k2/1 -> Product3/1
  "[2]^4"/1(Out1) -> Product3/2
  "[2]^3"/1(Out1) -> Product2/2
  Product3/1 -> Sum3/1
  Sum4/1 -> Integrator2/1
  k3/1 -> Product5/1
  "[2]^6"/1(Out1) -> Product5/2
  ka3/1 -> Product4/1
  Add/1 -> BIG/1, "[2]^6"/2(In2), "[2]^5"/2(In2), "[2]^4"/2(In2), "[2]^3"/2(In2), "[2]^2"/2(In2), "[2]^1"/2(In2)
  "[2]^5"/1(Out1) -> Product4/2
  Product5/1 -> Sum4/2
  Product4/1 -> Sum4/1
  BIG/1 -> Sum4/3
  Product2/1 -> Sum5/1
  Sum5/1 -> Sum2/2
  u/1 -> Sum5/2
  Constant/1 -> "[2]^1"/1(In1)
  Constant1/1 -> "[2]^2"/1(beta1)
  Constant2/1 -> "[2]^3"/1(In1)
  Constant3/1 -> "[2]^4"/1(beta1)
  Constant4/1 -> "[2]^5"/1(In1)
  Constant5/1 -> "[2]^6"/1(beta1)

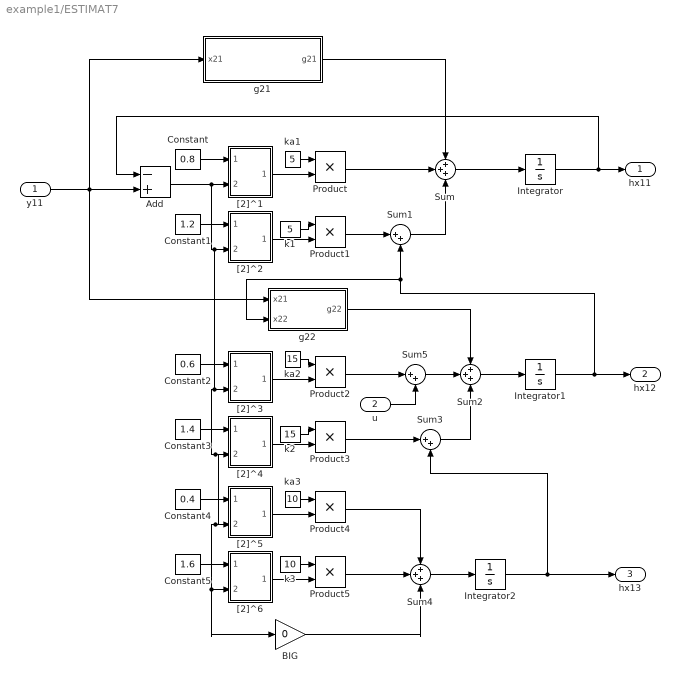
== system example1/ESTIMAT7 ==
  y11 : Inport
  u : Inport  Port=2
  Add : Sum  Inputs=-+
  BIG : Gain  Gain=0
  Constant : Constant  Value=0.8
  Constant1 : Constant  Value=1.2
  Constant2 : Constant  Value=0.6
  Constant3 : Constant  Value=1.4
  Constant4 : Constant  Value=0.4
  Constant5 : Constant  Value=1.6
  Integrator : Integrator  InitialCondition=1
  Integrator1 : Integrator  InitialCondition=1
  Integrator2 : Integrator  InitialCondition=1
  Product{,1..5} (6 alike) : Product
  Sum : Sum  Inputs=3
  Sum1 : Sum  Inputs=|++
  Sum2 : Sum  Inputs=3
  Sum3 : Sum  Inputs=|++
  Sum4 : Sum  Inputs=3
  Sum5 : Sum  Inputs=|++
  "[2]^1" : Subsystem
  "[2]^2" : Subsystem
  "[2]^3" : Subsystem
  "[2]^4" : Subsystem
  "[2]^5" : Subsystem
  "[2]^6" : Subsystem
  g21 : Subsystem
  g22 : Subsystem
  k1 : Constant  Value=5
  k2 : Constant  Value=15
  k3 : Constant  Value=10
  ka1 : Constant  Value=5
  ka2 : Constant  Value=15
  ka3 : Constant  Value=10
  hx11 : Outport
  hx12 : Outport  Port=2
  hx13 : Outport  Port=3
  wires:
  Integrator/1 -> Add/1, hx11/1
  Sum1/1 -> Sum/3
  Sum/1 -> Integrator/1
  Integrator1/1 -> g22/2(x22), Sum1/2, hx12/1
  y11/1 -> g22/1(x21), g21/1(x21), Add/2
  "[2]^1"/1(Out1) -> Product/2
  "[2]^2"/1(Out1) -> Product1/2
  ka1/1 -> Product/1
  k1/1 -> Product1/1
  g21/1(g21) -> Sum/1
  Product/1 -> Sum/2
  Product1/1 -> Sum1/1
  Sum2/1 -> Integrator1/1
  Sum3/1 -> Sum2/3
  Integrator2/1 -> hx13/1, Sum3/2
  g22/1(g22) -> Sum2/1
  ka2/1 -> Product2/1
  k2/1 -> Product3/1
  "[2]^4"/1(Out1) -> Product3/2
  "[2]^3"/1(Out1) -> Product2/2
  Product3/1 -> Sum3/1
  Sum4/1 -> Integrator2/1
  k3/1 -> Product5/1
  "[2]^6"/1(Out1) -> Product5/2
  ka3/1 -> Product4/1
  Add/1 -> BIG/1, "[2]^6"/2(In2), "[2]^5"/2(In2), "[2]^4"/2(In2), "[2]^3"/2(In2), "[2]^2"/2(In2), "[2]^1"/2(In2)
  "[2]^5"/1(Out1) -> Product4/2
  Product5/1 -> Sum4/2
  Product4/1 -> Sum4/1
  BIG/1 -> Sum4/3
  Product2/1 -> Sum5/1
  Sum5/1 -> Sum2/2
  u/1 -> Sum5/2
  Constant/1 -> "[2]^1"/1(In1)
  Constant1/1 -> "[2]^2"/1(beta1)
  Constant2/1 -> "[2]^3"/1(In1)
  Constant3/1 -> "[2]^4"/1(beta1)
  Constant4/1 -> "[2]^5"/1(In1)
  Constant5/1 -> "[2]^6"/1(beta1)

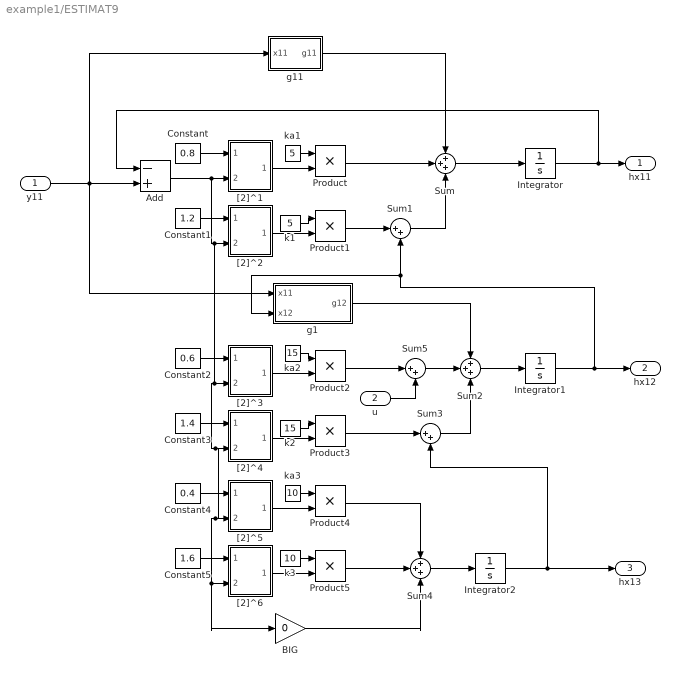
== system example1/ESTIMAT9 ==
  y11 : Inport
  u : Inport  Port=2
  Add : Sum  Inputs=-+
  BIG : Gain  Gain=0
  Constant : Constant  Value=0.8
  Constant1 : Constant  Value=1.2
  Constant2 : Constant  Value=0.6
  Constant3 : Constant  Value=1.4
  Constant4 : Constant  Value=0.4
  Constant5 : Constant  Value=1.6
  Integrator : Integrator  InitialCondition=1
  Integrator1 : Integrator  InitialCondition=1
  Integrator2 : Integrator  InitialCondition=1
  Product{,1..5} (6 alike) : Product
  Sum : Sum  Inputs=3
  Sum1 : Sum  Inputs=|++
  Sum2 : Sum  Inputs=3
  Sum3 : Sum  Inputs=|++
  Sum4 : Sum  Inputs=3
  Sum5 : Sum  Inputs=|++
  "[2]^1" : Subsystem
  "[2]^2" : Subsystem
  "[2]^3" : Subsystem
  "[2]^4" : Subsystem
  "[2]^5" : Subsystem
  "[2]^6" : Subsystem
  g1 : Subsystem
  g11 : Subsystem
  k1 : Constant  Value=5
  k2 : Constant  Value=15
  k3 : Constant  Value=10
  ka1 : Constant  Value=5
  ka2 : Constant  Value=15
  ka3 : Constant  Value=10
  hx11 : Outport
  hx12 : Outport  Port=2
  hx13 : Outport  Port=3
  wires:
  Integrator/1 -> Add/1, hx11/1
  Sum1/1 -> Sum/3
  Sum/1 -> Integrator/1
  Integrator1/1 -> g1/2(x12), Sum1/2, hx12/1
  y11/1 -> g1/1(x11), g11/1(x11), Add/2
  "[2]^1"/1(Out1) -> Product/2
  "[2]^2"/1(Out1) -> Product1/2
  ka1/1 -> Product/1
  k1/1 -> Product1/1
  g11/1(g11) -> Sum/1
  Product/1 -> Sum/2
  Product1/1 -> Sum1/1
  Sum2/1 -> Integrator1/1
  Sum3/1 -> Sum2/3
  Integrator2/1 -> hx13/1, Sum3/2
  g1/1(g12) -> Sum2/1
  ka2/1 -> Product2/1
  k2/1 -> Product3/1
  "[2]^4"/1(Out1) -> Product3/2
  "[2]^3"/1(Out1) -> Product2/2
  Product3/1 -> Sum3/1
  Sum4/1 -> Integrator2/1
  k3/1 -> Product5/1
  "[2]^6"/1(Out1) -> Product5/2
  ka3/1 -> Product4/1
  Add/1 -> BIG/1, "[2]^6"/2(In2), "[2]^5"/2(In2), "[2]^4"/2(In2), "[2]^3"/2(In2), "[2]^2"/2(In2), "[2]^1"/2(In2)
  "[2]^5"/1(Out1) -> Product4/2
  Product5/1 -> Sum4/2
  Product4/1 -> Sum4/1
  BIG/1 -> Sum4/3
  Product2/1 -> Sum5/1
  Sum5/1 -> Sum2/2
  u/1 -> Sum5/2
  Constant/1 -> "[2]^1"/1(In1)
  Constant1/1 -> "[2]^2"/1(beta1)
  Constant2/1 -> "[2]^3"/1(In1)
  Constant3/1 -> "[2]^4"/1(beta1)
  Constant4/1 -> "[2]^5"/1(In1)
  Constant5/1 -> "[2]^6"/1(beta1)

== system example1/SYSTEM1 ==
  u1 : Inport
  t : Inport  Port=2
  Integrator : Integrator  InitialCondition=15
  Integrator1 : Integrator  InitialCondition=5
  Sum : Sum  Inputs=|++
  Sum1 : Sum  Inputs=3
  f1 : Subsystem
  g11 : Subsystem
  g12 : Subsystem
  x11 : Outport
  x12 : Outport  Port=2
  f : Outport  Port=3
  wires:
  Integrator/1 -> g11/1(x11), f1/3(x1), g12/1(x11), x11/1
  Sum/1 -> Integrator/1
  g11/1(g11) -> Sum/1
  Integrator1/1 -> x12/1, Sum/2, f1/2(x2), g12/2(x12)
  Sum1/1 -> Integrator1/1
  u1/1 -> Sum1/2
  g12/1(g12) -> Sum1/1
  f1/1(f) -> Sum1/3, f/1
  t/1 -> f1/1(t)

== system example1/SYSTEM2 ==
  u2 : Inport
  t : Inport  Port=2
  Integrator : Integrator  InitialCondition=1
  Integrator1 : Integrator  InitialCondition=-1
  Sum : Sum  Inputs=|++
  Sum1 : Sum  Inputs=3
  f2 : Subsystem
  g21 : Subsystem
  g22 : Subsystem
  x21 : Outport
  x22 : Outport  Port=2
  f : Outport  Port=3
  wires:
  Integrator/1 -> f2/2(x1), g22/1(x21), g21/1(x21), x21/1
  Integrator1/1 -> x22/1, g22/2(x22), Sum/2
  Sum/1 -> Integrator/1
  g21/1(g21) -> Sum/1
  Sum1/1 -> Integrator1/1
  u2/1 -> Sum1/2
  g22/1(g22) -> Sum1/1
  f2/1(f2) -> f/1, Sum1/3
  t/1 -> f2/1(t)

== system example1/SYSTEM3 ==
  u1 : Inport
  t : Inport  Port=2
  Integrator : Integrator  InitialCondition=15
  Integrator1 : Integrator  InitialCondition=5
  Sum : Sum  Inputs=|++
  Sum1 : Sum  Inputs=3
  f1 : Subsystem
  g11 : Subsystem
  g12 : Subsystem
  x11 : Outport
  x12 : Outport  Port=2
  f : Outport  Port=3
  wires:
  Integrator/1 -> f1/2(x1), g12/1(x11), g11/1(x11), x11/1
  Sum/1 -> Integrator/1
  g11/1(g11) -> Sum/1
  Integrator1/1 -> x12/1, Sum/2, g12/2(x12), f1/3(x2)
  Sum1/1 -> Integrator1/1
  u1/1 -> Sum1/2
  g12/1(g12) -> Sum1/1
  f1/1(f) -> Sum1/3, f/1
  t/1 -> f1/1(t)

== system example1/SYSTEM4 ==
  u2 : Inport
  t : Inport  Port=2
  Integrator : Integrator  InitialCondition=1
  Integrator1 : Integrator  InitialCondition=-1
  Sum : Sum  Inputs=|++
  Sum1 : Sum  Inputs=3
  f2 : Subsystem
  g21 : Subsystem
  g22 : Subsystem
  x21 : Outport
  x22 : Outport  Port=2
  f : Outport  Port=3
  wires:
  Integrator/1 -> f2/2(x1), g22/1(x21), g21/1(x21), x21/1
  Integrator1/1 -> x22/1, f2/3(x2), g22/2(x22), Sum/2
  Sum/1 -> Integrator/1
  g21/1(g21) -> Sum/1
  Sum1/1 -> Integrator1/1
  u2/1 -> Sum1/2
  g22/1(g22) -> Sum1/1
  f2/1(f2) -> f/1, Sum1/3
  t/1 -> f2/1(t)

== system example1/SYSTEM5 ==
  u1 : Inport
  t : Inport  Port=2
  Integrator : Integrator  InitialCondition=25
  Integrator1 : Integrator  InitialCondition=5
  Sum : Sum  Inputs=|++
  Sum1 : Sum  Inputs=3
  f1 : Subsystem
  g11 : Subsystem
  g12 : Subsystem
  x11 : Outport
  x12 : Outport  Port=2
  f : Outport  Port=3
  wires:
  Integrator/1 -> g11/1(x11), f1/3(x1), g12/1(x11), x11/1
  Sum/1 -> Integrator/1
  g11/1(g11) -> Sum/1
  Integrator1/1 -> x12/1, Sum/2, f1/2(x2), g12/2(x12)
  Sum1/1 -> Integrator1/1
  u1/1 -> Sum1/2
  g12/1(g12) -> Sum1/1
  f1/1(f) -> Sum1/3, f/1
  t/1 -> f1/1(t)

== system example1/SYSTEM6 ==
  u2 : Inport
  t : Inport  Port=2
  Integrator : Integrator  InitialCondition=25
  Integrator1 : Integrator  InitialCondition=-1
  Sum : Sum  Inputs=|++
  Sum1 : Sum  Inputs=3
  f2 : Subsystem
  g21 : Subsystem
  g22 : Subsystem
  x21 : Outport
  x22 : Outport  Port=2
  f : Outport  Port=3
  wires:
  Integrator/1 -> f2/2(x1), g22/1(x21), g21/1(x21), x21/1
  Integrator1/1 -> x22/1, g22/2(x22), Sum/2
  Sum/1 -> Integrator/1
  g21/1(g21) -> Sum/1
  Sum1/1 -> Integrator1/1
  u2/1 -> Sum1/2
  g22/1(g22) -> Sum1/1
  f2/1(f2) -> f/1, Sum1/3
  t/1 -> f2/1(t)

== system example1/SYSTEM7 ==
  u1 : Inport
  t : Inport  Port=2
  Integrator : Integrator  InitialCondition=40
  Integrator1 : Integrator  InitialCondition=5
  Sum : Sum  Inputs=|++
  Sum1 : Sum  Inputs=3
  f1 : Subsystem
  g11 : Subsystem
  g12 : Subsystem
  x11 : Outport
  x12 : Outport  Port=2
  f : Outport  Port=3
  wires:
  Integrator/1 -> f1/2(x1), g12/1(x11), g11/1(x11), x11/1
  Sum/1 -> Integrator/1
  g11/1(g11) -> Sum/1
  Integrator1/1 -> x12/1, Sum/2, f1/3(x2), g12/2(x12)
  Sum1/1 -> Integrator1/1
  u1/1 -> Sum1/2
  g12/1(g12) -> Sum1/1
  f1/1(f) -> Sum1/3, f/1
  t/1 -> f1/1(t)

== system example1/SYSTEM8 ==
  u2 : Inport
  t : Inport  Port=2
  Integrator : Integrator  InitialCondition=25
  Integrator1 : Integrator  InitialCondition=-1
  Sum : Sum  Inputs=|++
  Sum1 : Sum  Inputs=3
  f2 : Subsystem
  g21 : Subsystem
  g22 : Subsystem
  x21 : Outport
  x22 : Outport  Port=2
  f : Outport  Port=3
  wires:
  Integrator/1 -> f2/2(x1), g22/1(x21), g21/1(x21), x21/1
  Integrator1/1 -> x22/1, f2/3(x2), g22/2(x22), Sum/2
  Sum/1 -> Integrator/1
  g21/1(g21) -> Sum/1
  Sum1/1 -> Integrator1/1
  u2/1 -> Sum1/2
  g22/1(g22) -> Sum1/1
  f2/1(f2) -> f/1, Sum1/3
  t/1 -> f2/1(t)

== system example1/Subsystem1 ==
  c1 : Inport
  c2 : Inport  Port=2
  p/q : Inport  Port=3
  s2 : Inport  Port=4
  alpha2 : Inport  Port=5
  x21 : Inport  Port=6
  hx22 : Inport  Port=7
  hx23 : Inport  Port=8
  Add : Sum  Inputs=-+
  Add1 : Sum  Inputs=4
  Constant : Constant  Value=2
  Gain : Gain  Gain=-1
  Gain1 : Gain  Gain=-1
  Gain2 : Gain  Gain=-1
  Pow : Math  Operator=pow  SignedPower=on  RndMeth=Zero
  Pow1 : Math  Operator=pow  SignedPower=on  RndMeth=Zero
  Product : Product
  Product1 : Product
  SAT : Subsystem  Commented=through
  Scope : Scope
  Subsystem : Subsystem
  Sum : Sum  Inputs=|+-
  Sum1 : Sum  Inputs=|+-
  g1 : Subsystem
  u2 : Outport
  wires:
  p/q/1 -> Pow1/2, Add/1
  Constant/1 -> Add/2
  s2/1 -> Gain2/1, Pow1/1, Pow/1
  Add/1 -> Pow/2
  Pow/1 -> Gain/1
  Pow1/1 -> Gain1/1
  Gain/1 -> Product/2
  c1/1 -> Product/1
  Gain1/1 -> Product1/1
  c2/1 -> Product1/2
  alpha2/1 -> Subsystem/1(alpha)
  Product/1 -> Add1/1
  Product1/1 -> Add1/2
  Gain2/1 -> Add1/3
  Subsystem/2(tao2) -> Scope/1, Add1/4
  Add1/1 -> Sum/1
  x21/1 -> g1/1(x21)
  hx22/1 -> g1/2(x22)
  g1/1(g22) -> Sum/2
  Sum/1 -> Sum1/1
  hx23/1 -> Sum1/2
  Sum1/1 -> SAT/1(In1)
  SAT/1(u1) -> u2/1

== system example1/Subsystem10 ==
  c1 : Inport
  c2 : Inport  Port=2
  p/q : Inport  Port=3
  s2 : Inport  Port=4
  alpha2 : Inport  Port=5
  x21 : Inport  Port=6
  hx22 : Inport  Port=7
  hx23 : Inport  Port=8
  Add : Sum  Inputs=-+
  Add1 : Sum  Inputs=4
  Constant : Constant  Value=2
  Gain : Gain  Gain=-1
  Gain1 : Gain  Gain=-1
  Gain2 : Gain  Gain=-1
  Pow : Math  Operator=pow  SignedPower=on  RndMeth=Zero
  Pow1 : Math  Operator=pow  SignedPower=on  RndMeth=Zero
  Product : Product
  Product1 : Product
  SAT : Subsystem  Commented=through
  Subsystem : Subsystem
  Sum : Sum  Inputs=|+-
  Sum1 : Sum  Inputs=|+-
  g22 : Subsystem
  u2 : Outport
  wires:
  p/q/1 -> Pow1/2, Add/1
  Constant/1 -> Add/2
  s2/1 -> Gain2/1, Pow1/1, Pow/1
  Add/1 -> Pow/2
  Pow/1 -> Gain/1
  Pow1/1 -> Gain1/1
  Gain/1 -> Product/2
  c1/1 -> Product/1
  Gain1/1 -> Product1/1
  c2/1 -> Product1/2
  alpha2/1 -> Subsystem/1(alpha)
  Product/1 -> Add1/1
  Product1/1 -> Add1/2
  Gain2/1 -> Add1/3
  Subsystem/2(tao2) -> Add1/4
  Add1/1 -> Sum/1
  x21/1 -> g22/1(x21)
  hx22/1 -> g22/2(x22)
  g22/1(g22) -> Sum/2
  Sum/1 -> Sum1/1
  hx23/1 -> Sum1/2
  Sum1/1 -> SAT/1(In1)
  SAT/1(u1) -> u2/1

== system example1/Subsystem11 ==
  hx22 : Inport
  alpha2 : Inport  Port=2
  Add : Sum  Inputs=+-
  s2 : Outport
  wires:
  hx22/1 -> Add/1
  alpha2/1 -> Add/2
  Add/1 -> s2/1

== system example1/Subsystem12 ==
  hx32 : Inport
  alpha3 : Inport  Port=2
  Add : Sum  Inputs=+-
  Scope : Scope
  s3 : Outport
  wires:
  hx32/1 -> Add/1
  alpha3/1 -> Scope/1, Add/2
  Add/1 -> s3/1

== system example1/Subsystem13 ==
  hx42 : Inport
  alpha4 : Inport  Port=2
  Add : Sum  Inputs=+-
  s4 : Outport
  wires:
  hx42/1 -> Add/1
  alpha4/1 -> Add/2
  Add/1 -> s4/1

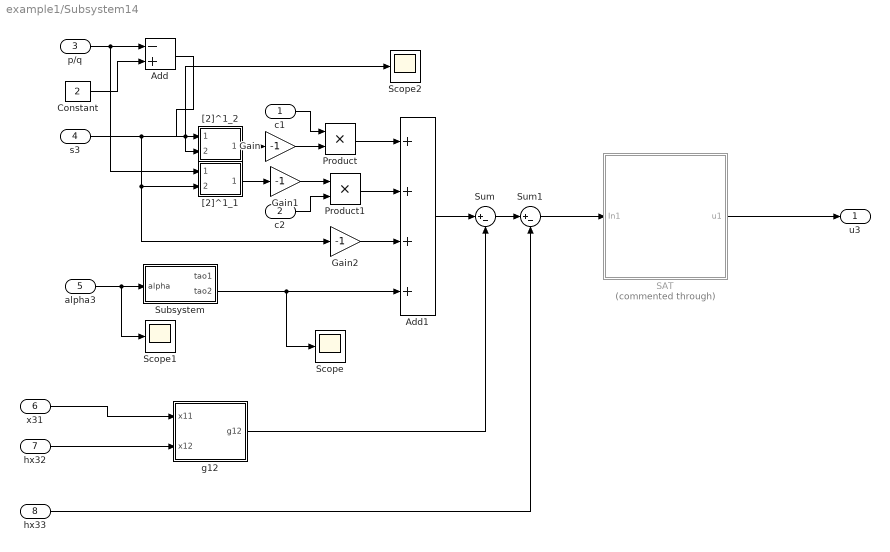
== system example1/Subsystem14 ==
  c1 : Inport
  c2 : Inport  Port=2
  p/q : Inport  Port=3
  s3 : Inport  Port=4
  alpha3 : Inport  Port=5
  x31 : Inport  Port=6
  hx32 : Inport  Port=7
  hx33 : Inport  Port=8
  Add : Sum  Inputs=-+
  Add1 : Sum  Inputs=4
  Constant : Constant  Value=2
  Gain : Gain  Gain=-1
  Gain1 : Gain  Gain=-1
  Gain2 : Gain  Gain=-1
  Product : Product
  Product1 : Product
  SAT : Subsystem  Commented=through
  Scope : Scope
  Scope1 : Scope
  Scope2 : Scope
  Subsystem : Subsystem
  Sum : Sum  Inputs=|+-
  Sum1 : Sum  Inputs=|+-
  "[2]^1_1" : Subsystem
  "[2]^1_2" : Subsystem
  g12 : Subsystem
  u3 : Outport
  wires:
  p/q/1 -> "[2]^1_1"/1(p/q), Add/1
  Constant/1 -> Add/2
  s3/1 -> "[2]^1_2"/2(2), Scope2/1, Gain2/1, "[2]^1_1"/2(2)
  Add/1 -> "[2]^1_2"/1(In1)
  "[2]^1_2"/1(Out1) -> Gain/1
  "[2]^1_1"/1(Out1) -> Gain1/1
  Gain/1 -> Product/2
  c1/1 -> Product/1
  Gain1/1 -> Product1/1
  c2/1 -> Product1/2
  alpha3/1 -> Scope1/1, Subsystem/1(alpha)
  Product/1 -> Add1/1
  Product1/1 -> Add1/2
  Gain2/1 -> Add1/3
  Subsystem/2(tao2) -> Scope/1, Add1/4
  Add1/1 -> Sum/1
  x31/1 -> g12/1(x11)
  hx32/1 -> g12/2(x12)
  Sum/1 -> Sum1/1
  g12/1(g12) -> Sum/2
  hx33/1 -> Sum1/2
  Sum1/1 -> SAT/1(In1)
  SAT/1(u1) -> u3/1

== system example1/Subsystem15 ==
  c1 : Inport
  c2 : Inport  Port=2
  p/q : Inport  Port=3
  s4 : Inport  Port=4
  alpha4 : Inport  Port=5
  x41 : Inport  Port=6
  hx42 : Inport  Port=7
  hx43 : Inport  Port=8
  Add : Sum  Inputs=-+
  Add1 : Sum  Inputs=4
  Constant : Constant  Value=2
  Gain : Gain  Gain=-1
  Gain1 : Gain  Gain=-1
  Gain2 : Gain  Gain=-1
  Pow : Math  Operator=pow  SignedPower=on  RndMeth=Zero
  Pow1 : Math  Operator=pow  SignedPower=on  RndMeth=Zero
  Product : Product
  Product1 : Product
  SAT : Subsystem  Commented=through
  Subsystem : Subsystem
  Sum : Sum  Inputs=|+-
  Sum1 : Sum  Inputs=|+-
  g22 : Subsystem
  u4 : Outport
  wires:
  p/q/1 -> Pow1/2, Add/1
  Constant/1 -> Add/2
  s4/1 -> Gain2/1, Pow1/1, Pow/1
  Add/1 -> Pow/2
  Pow/1 -> Gain/1
  Pow1/1 -> Gain1/1
  Gain/1 -> Product/2
  c1/1 -> Product/1
  Gain1/1 -> Product1/1
  c2/1 -> Product1/2
  alpha4/1 -> Subsystem/1(alpha)
  Product/1 -> Add1/1
  Product1/1 -> Add1/2
  Gain2/1 -> Add1/3
  Subsystem/2(tao2) -> Add1/4
  Add1/1 -> Sum/1
  Sum/1 -> Sum1/1
  hx42/1 -> g22/2(x22)
  x41/1 -> g22/1(x21)
  g22/1(g22) -> Sum/2
  hx43/1 -> Sum1/2
  Sum1/1 -> SAT/1(In1)
  SAT/1(u1) -> u4/1

== system example1/Subsystem16 ==
  hx42 : Inport
  alpha4 : Inport  Port=2
  Add : Sum  Inputs=+-
  s4 : Outport
  wires:
  hx42/1 -> Add/1
  alpha4/1 -> Add/2
  Add/1 -> s4/1

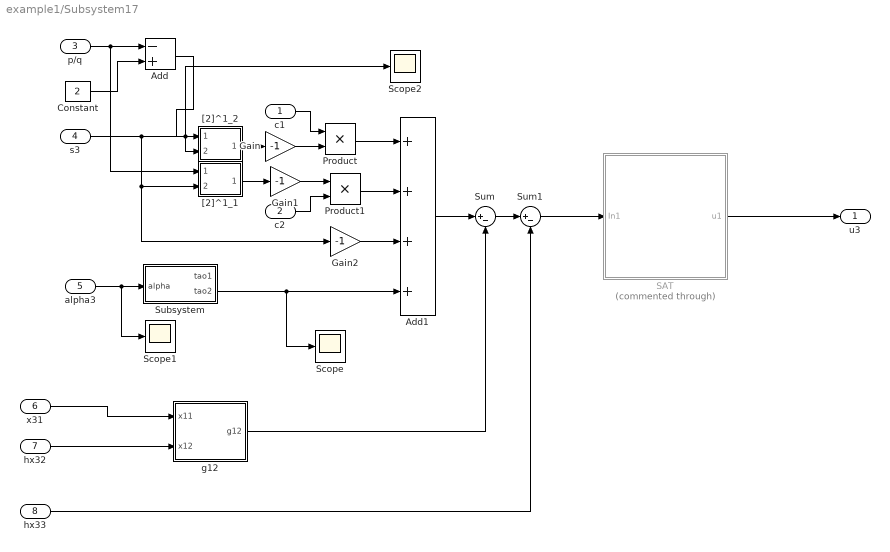
== system example1/Subsystem17 ==
  c1 : Inport
  c2 : Inport  Port=2
  p/q : Inport  Port=3
  s3 : Inport  Port=4
  alpha3 : Inport  Port=5
  x31 : Inport  Port=6
  hx32 : Inport  Port=7
  hx33 : Inport  Port=8
  Add : Sum  Inputs=-+
  Add1 : Sum  Inputs=4
  Constant : Constant  Value=2
  Gain : Gain  Gain=-1
  Gain1 : Gain  Gain=-1
  Gain2 : Gain  Gain=-1
  Product : Product
  Product1 : Product
  SAT : Subsystem  Commented=through
  Scope : Scope
  Scope1 : Scope
  Scope2 : Scope
  Subsystem : Subsystem
  Sum : Sum  Inputs=|+-
  Sum1 : Sum  Inputs=|+-
  "[2]^1_1" : Subsystem
  "[2]^1_2" : Subsystem
  g12 : Subsystem
  u3 : Outport
  wires:
  p/q/1 -> "[2]^1_1"/1(p/q), Add/1
  Constant/1 -> Add/2
  s3/1 -> "[2]^1_2"/2(2), Scope2/1, Gain2/1, "[2]^1_1"/2(2)
  Add/1 -> "[2]^1_2"/1(In1)
  "[2]^1_2"/1(Out1) -> Gain/1
  "[2]^1_1"/1(Out1) -> Gain1/1
  Gain/1 -> Product/2
  c1/1 -> Product/1
  Gain1/1 -> Product1/1
  c2/1 -> Product1/2
  alpha3/1 -> Scope1/1, Subsystem/1(alpha)
  Product/1 -> Add1/1
  Product1/1 -> Add1/2
  Gain2/1 -> Add1/3
  Subsystem/2(tao2) -> Scope/1, Add1/4
  Add1/1 -> Sum/1
  x31/1 -> g12/1(x11)
  hx32/1 -> g12/2(x12)
  Sum/1 -> Sum1/1
  g12/1(g12) -> Sum/2
  hx33/1 -> Sum1/2
  Sum1/1 -> SAT/1(In1)
  SAT/1(u1) -> u3/1

== system example1/Subsystem18 ==
  c1 : Inport
  c2 : Inport  Port=2
  p/q : Inport  Port=3
  s4 : Inport  Port=4
  alpha4 : Inport  Port=5
  x41 : Inport  Port=6
  hx42 : Inport  Port=7
  hx43 : Inport  Port=8
  Add : Sum  Inputs=-+
  Add1 : Sum  Inputs=4
  Constant : Constant  Value=2
  Gain : Gain  Gain=-1
  Gain1 : Gain  Gain=-1
  Gain2 : Gain  Gain=-1
  Pow : Math  Operator=pow  SignedPower=on  RndMeth=Zero
  Pow1 : Math  Operator=pow  SignedPower=on  RndMeth=Zero
  Product : Product
  Product1 : Product
  SAT : Subsystem  Commented=through
  Subsystem : Subsystem
  Sum : Sum  Inputs=|+-
  Sum1 : Sum  Inputs=|+-
  g22 : Subsystem
  u4 : Outport
  wires:
  p/q/1 -> Pow1/2, Add/1
  Constant/1 -> Add/2
  s4/1 -> Gain2/1, Pow1/1, Pow/1
  Add/1 -> Pow/2
  Pow/1 -> Gain/1
  Pow1/1 -> Gain1/1
  Gain/1 -> Product/2
  c1/1 -> Product/1
  Gain1/1 -> Product1/1
  c2/1 -> Product1/2
  alpha4/1 -> Subsystem/1(alpha)
  Product/1 -> Add1/1
  Product1/1 -> Add1/2
  Gain2/1 -> Add1/3
  Subsystem/2(tao2) -> Add1/4
  Add1/1 -> Sum/1
  Sum/1 -> Sum1/1
  hx42/1 -> g22/2(x22)
  x41/1 -> g22/1(x21)
  g22/1(g22) -> Sum/2
  hx43/1 -> Sum1/2
  Sum1/1 -> SAT/1(In1)
  SAT/1(u1) -> u4/1

== system example1/Subsystem19 ==
  x11 : Inport
  SUMj-i : Inport  Port=2
  Add1 : Sum  Inputs=-+
  Add2 : Sum
  Gain : Gain  Gain=-1
  Integrator : Integrator
  Scope : Scope
  d : Constant  Value=45
  e1 : Outport
  wires:
  d/1 -> Add1/1
  x11/1 -> Add1/2
  SUMj-i/1 -> Integrator/1
  Integrator/1 -> Gain/1
  Gain/1 -> Add2/2
  Add1/1 -> Scope/1, Add2/1
  Add2/1 -> e1/1

== system example1/Subsystem2 ==
  hx22 : Inport
  alpha2 : Inport  Port=2
  Add : Sum  Inputs=+-
  s2 : Outport
  wires:
  hx22/1 -> Add/1
  alpha2/1 -> Add/2
  Add/1 -> s2/1

== system example1/Subsystem20 ==
  x21 : Inport
  SUMj-i : Inport  Port=2
  Add1 : Sum  Inputs=-+
  Add2 : Sum
  Gain : Gain  Gain=-1
  Integrator : Integrator
  di : Constant  Value=40
  e2 : Outport
  wires:
  di/1 -> Add1/1
  x21/1 -> Add1/2
  SUMj-i/1 -> Integrator/1
  Integrator/1 -> Gain/1
  Gain/1 -> Add2/2
  Add1/1 -> Add2/1
  Add2/1 -> e2/1

== system example1/Subsystem21 ==
  x31 : Inport
  SUMj-i : Inport  Port=2
  Add1 : Sum  Inputs=-+
  Add2 : Sum
  Gain : Gain  Gain=-1
  Integrator : Integrator
  di : Constant  Value=25
  e3 : Outport
  wires:
  di/1 -> Add1/1
  x31/1 -> Add1/2
  SUMj-i/1 -> Integrator/1
  Integrator/1 -> Gain/1
  Gain/1 -> Add2/2
  Add1/1 -> Add2/1
  Add2/1 -> e3/1

== system example1/Subsystem22 ==
  x41 : Inport
  SUMj-i : Inport  Port=2
  Add1 : Sum  Inputs=-+
  Add2 : Sum
  Gain : Gain  Gain=-1
  Integrator : Integrator
  di : Constant  Value=35
  e4 : Outport
  wires:
  di/1 -> Add1/1
  x41/1 -> Add1/2
  SUMj-i/1 -> Integrator/1
  Integrator/1 -> Gain/1
  Gain/1 -> Add2/2
  Add1/1 -> Add2/1
  Add2/1 -> e4/1

== system example1/Subsystem23 ==
  hx12 : Inport
  alpha1 : Inport  Port=2
  Add : Sum  Inputs=+-
  Scope : Scope
  s1 : Outport
  wires:
  hx12/1 -> Add/1
  alpha1/1 -> Add/2
  Add/1 -> Scope/1, s1/1

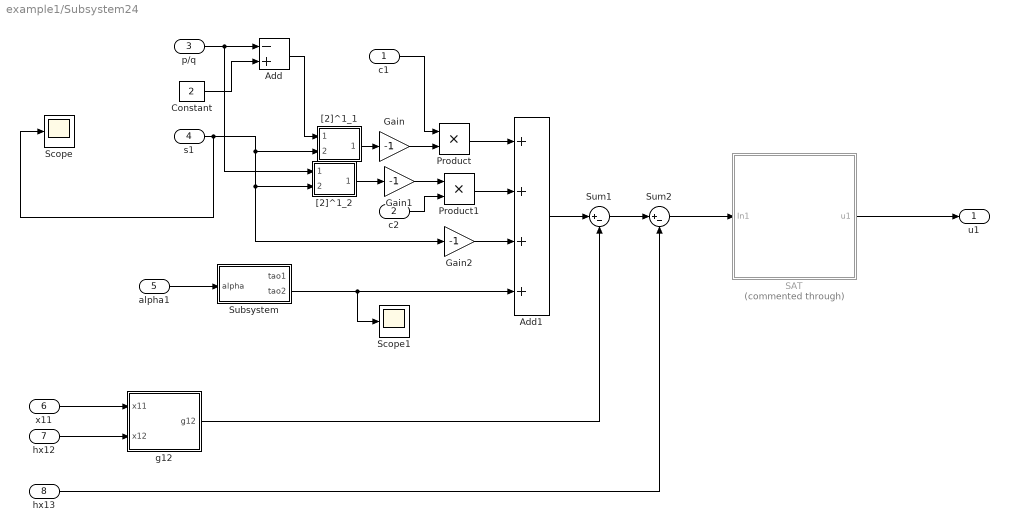
== system example1/Subsystem24 ==
  c1 : Inport
  c2 : Inport  Port=2
  p/q : Inport  Port=3
  s1 : Inport  Port=4
  alpha1 : Inport  Port=5
  x11 : Inport  Port=6
  hx12 : Inport  Port=7
  hx13 : Inport  Port=8
  Add : Sum  Inputs=-+
  Add1 : Sum  Inputs=4
  Constant : Constant  Value=2
  Gain : Gain  Gain=-1
  Gain1 : Gain  Gain=-1
  Gain2 : Gain  Gain=-1
  Product : Product
  Product1 : Product
  SAT : Subsystem  Commented=through
  Scope : Scope
  Scope1 : Scope
  Subsystem : Subsystem
  Sum1 : Sum  Inputs=|+-
  Sum2 : Sum  Inputs=|+-
  "[2]^1_1" : Subsystem
  "[2]^1_2" : Subsystem
  g12 : Subsystem
  u1 : Outport
  wires:
  p/q/1 -> "[2]^1_2"/1(p/q), Add/1
  Constant/1 -> Add/2
  s1/1 -> Scope/1, Gain2/1, "[2]^1_2"/2(2), "[2]^1_1"/2(2)
  Add/1 -> "[2]^1_1"/1(In1)
  "[2]^1_1"/1(Out1) -> Gain/1
  "[2]^1_2"/1(Out1) -> Gain1/1
  Gain/1 -> Product/2
  c1/1 -> Product/1
  Gain1/1 -> Product1/1
  c2/1 -> Product1/2
  alpha1/1 -> Subsystem/1(alpha)
  Product/1 -> Add1/1
  Product1/1 -> Add1/2
  Gain2/1 -> Add1/3
  Add1/1 -> Sum1/1
  Subsystem/2(tao2) -> Scope1/1, Add1/4
  g12/1(g12) -> Sum1/2
  x11/1 -> g12/1(x11)
  hx12/1 -> g12/2(x12)
  Sum1/1 -> Sum2/1
  hx13/1 -> Sum2/2
  Sum2/1 -> SAT/1(In1)
  SAT/1(u1) -> u1/1

== system example1/Subsystem3 ==
  hx32 : Inport
  alpha3 : Inport  Port=2
  Add : Sum  Inputs=+-
  Scope : Scope
  s3 : Outport
  wires:
  hx32/1 -> Add/1
  alpha3/1 -> Scope/1, Add/2
  Add/1 -> s3/1

== system example1/Subsystem4 ==
  x11 : Inport
  SUMj-i : Inport  Port=2
  Add1 : Sum  Inputs=-+
  Add2 : Sum
  Gain : Gain  Gain=-1
  Integrator : Integrator
  Scope : Scope
  d : Constant  Value=45
  e1 : Outport
  wires:
  d/1 -> Add1/1
  x11/1 -> Add1/2
  SUMj-i/1 -> Integrator/1
  Integrator/1 -> Gain/1
  Gain/1 -> Add2/2
  Add1/1 -> Scope/1, Add2/1
  Add2/1 -> e1/1

== system example1/Subsystem5 ==
  x21 : Inport
  SUMj-i : Inport  Port=2
  Add1 : Sum  Inputs=-+
  Add2 : Sum
  Gain : Gain  Gain=-1
  Integrator : Integrator
  di : Constant  Value=40
  e2 : Outport
  wires:
  di/1 -> Add1/1
  x21/1 -> Add1/2
  SUMj-i/1 -> Integrator/1
  Integrator/1 -> Gain/1
  Gain/1 -> Add2/2
  Add1/1 -> Add2/1
  Add2/1 -> e2/1

== system example1/Subsystem6 ==
  x31 : Inport
  SUMj-i : Inport  Port=2
  Add1 : Sum  Inputs=-+
  Add2 : Sum
  Gain : Gain  Gain=-1
  Integrator : Integrator
  di : Constant  Value=25
  e3 : Outport
  wires:
  di/1 -> Add1/1
  x31/1 -> Add1/2
  SUMj-i/1 -> Integrator/1
  Integrator/1 -> Gain/1
  Gain/1 -> Add2/2
  Add1/1 -> Add2/1
  Add2/1 -> e3/1

== system example1/Subsystem7 ==
  x41 : Inport
  SUMj-i : Inport  Port=2
  Add1 : Sum  Inputs=-+
  Add2 : Sum
  Gain : Gain  Gain=-1
  Integrator : Integrator
  di : Constant  Value=35
  e4 : Outport
  wires:
  di/1 -> Add1/1
  x41/1 -> Add1/2
  SUMj-i/1 -> Integrator/1
  Integrator/1 -> Gain/1
  Gain/1 -> Add2/2
  Add1/1 -> Add2/1
  Add2/1 -> e4/1

== system example1/Subsystem8 ==
  hx12 : Inport
  alpha1 : Inport  Port=2
  Add : Sum  Inputs=+-
  Scope : Scope
  s1 : Outport
  wires:
  hx12/1 -> Add/1
  alpha1/1 -> Add/2
  Add/1 -> Scope/1, s1/1

== system example1/Subsystem9 ==
  c1 : Inport
  c2 : Inport  Port=2
  p/q : Inport  Port=3
  s1 : Inport  Port=4
  alpha1 : Inport  Port=5
  x11 : Inport  Port=6
  hx12 : Inport  Port=7
  hx13 : Inport  Port=8
  Add : Sum  Inputs=-+
  Add1 : Sum  Inputs=4
  Constant : Constant  Value=2
  Gain : Gain  Gain=-1
  Gain1 : Gain  Gain=-1
  Gain2 : Gain  Gain=-1
  Product : Product
  Product1 : Product
  SAT : Subsystem  Commented=through
  Scope : Scope
  Scope1 : Scope
  Subsystem : Subsystem
  Sum1 : Sum  Inputs=|+-
  Sum2 : Sum  Inputs=|+-
  "[2]^1_1" : Subsystem
  "[2]^1_2" : Subsystem
  g12 : Subsystem
  u1 : Outport
  wires:
  p/q/1 -> "[2]^1_2"/1(p/q), Add/1
  Constant/1 -> Add/2
  s1/1 -> Scope/1, Gain2/1, "[2]^1_2"/2(2), "[2]^1_1"/2(2)
  Add/1 -> "[2]^1_1"/1(In1)
  "[2]^1_1"/1(Out1) -> Gain/1
  "[2]^1_2"/1(Out1) -> Gain1/1
  Gain/1 -> Product/2
  c1/1 -> Product/1
  Gain1/1 -> Product1/1
  c2/1 -> Product1/2
  alpha1/1 -> Subsystem/1(alpha)
  Product/1 -> Add1/1
  Product1/1 -> Add1/2
  Gain2/1 -> Add1/3
  Add1/1 -> Sum1/1
  Subsystem/2(tao2) -> Scope1/1, Add1/4
  g12/1(g12) -> Sum1/2
  x11/1 -> g12/1(x11)
  hx12/1 -> g12/2(x12)
  Sum1/1 -> Sum2/1
  hx13/1 -> Sum2/2
  Sum2/1 -> SAT/1(In1)
  SAT/1(u1) -> u1/1
